simulink model "EVX_Lap_Simulation"  (R2018b)
settings: Solver=FixedStepAuto  StartTime=0  StopTime=100  FixedStep=0.01  MinStep=0.001  RelTol=1e-3
undefined symbols (not defined in the file): Car, dist, DOD, initial_velocity, motorefficiency, motormaxtorque, motorspeedradps, R0model, theta_d, Track_Dist, velocity_dnew, VoltageDOD, x, y
libraries: simulink x4
(part 1 of 3)
settings Model: Creator=Foster  LastModifiedBy=wjfos
settings SolverCC: AlgebraicLoopSolver=LineSearch
settings DebuggingCC: UnderspecifiedInitializationDetection=Classic  MergeDetectMultiDrivingBlocksExec=warning  MaxConsecutiveZCsMsg=warning  FcnCallInpInsideContextMsg=warning  UnconnectedInputMsg=none  UnconnectedOutputMsg=none  UnconnectedLineMsg=none  ModelReferenceExtraNoncontSigs=warning  UnderSpecifiedDimensionMsg=warning
settings HardwareCC: ProdBitPerLong=64  ProdHWDeviceType=Intel->x86-64 (Mac OS X)

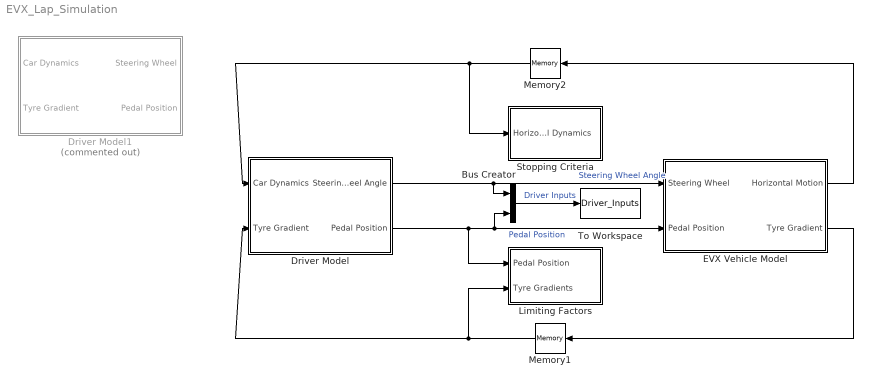
== system EVX_Lap_Simulation ==
  Bus Creator : BusCreator  Inputs=2
  Driver Model : Subsystem  Variant=on
  Driver Model1 : Subsystem  Commented=on
  EVX Vehicle Model : Subsystem
  Limiting Factors : Subsystem
  Memory1 : Memory  InheritSampleTime=on
  Memory2 : Memory  InheritSampleTime=on
  Stopping Criteria : Subsystem
  To Workspace : ToWorkspace  VariableName=Driver_Inputs  SaveFormat=Timeseries  SampleTime=-1
  wires:
  Driver Model/1(Steering Wheel Angle) -> Bus Creator/1, EVX Vehicle Model/1(Steering Wheel)  "Steering Wheel Angle"
  Driver Model/2(Pedal Position) -> Limiting Factors/1(Pedal Position), Bus Creator/2, EVX Vehicle Model/2(Pedal Position)  "Pedal Position"
  EVX Vehicle Model/1(Horizontal Motion) -> Memory2/1
  EVX Vehicle Model/2(Tyre Gradient) -> Memory1/1
  Memory1/1 -> Driver Model/2(Tyre Gradient), Limiting Factors/2(Tyre Gradients)
  Memory2/1 -> Driver Model/1(Car Dynamics), Stopping Criteria/1(Horizontal Dynamics)
  Bus Creator/1 -> To Workspace/1  "Driver Inputs"

== system EVX_Lap_Simulation/Driver Model ==
  Car Dynamics : Inport
  Tyre Gradient : Inport  Port=2
  Control System Driver Model : Subsystem  VariantControl=ControlSystemDriverModel
  Driver Input Model : Subsystem  VariantControl=InputDefinedDriverModel
  Steering Wheel Angle : Outport
  Pedal Position : Outport  Port=2

== system EVX_Lap_Simulation/Driver Model1 ==
  Car Dynamics : Inport
  Tyre Gradient : Inport  Port=2
  Control System Driver Model : Subsystem
  Driver Input Model : Subsystem
  Steering Wheel : Outport
  Pedal Position : Outport  Port=2

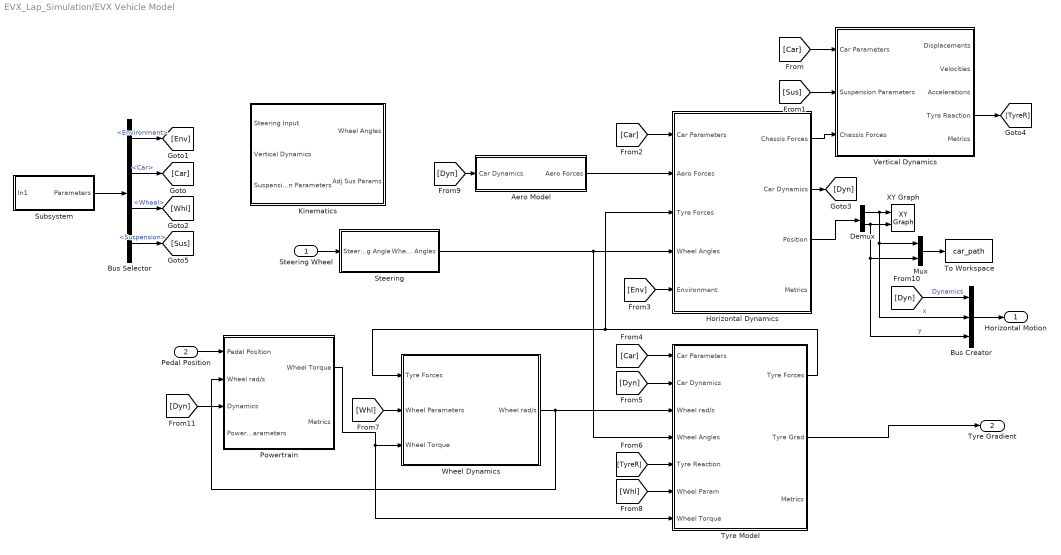
== system EVX_Lap_Simulation/EVX Vehicle Model ==
  Steering Wheel : Inport
  Pedal Position : Inport  Port=2
  Aero Model : Subsystem
  Bus Creator : BusCreator  Inputs=3
  Bus Selector : BusSelector  OutputSignals=Environment,Car,Wheel,Suspension
  Demux : Demux  Outputs=2
  Horizontal Dynamics : Subsystem
  Kinematics : Subsystem
  Mux : Mux  Inputs=2
  Powertrain : Subsystem
  Steering : Subsystem
  Subsystem : Subsystem
  To Workspace : ToWorkspace  VariableName=car_path  SaveFormat=Timeseries  SampleTime=-1
  Tyre Model : Subsystem
  Vertical Dynamics : Subsystem
  Wheel Dynamics : Subsystem
  XY Graph : simulink/Sinks/XY Graph  xmin=-400  xmax=100  ymin=-25  ymax=250  st=-1
  Horizontal Motion : Outport
  Tyre Gradient : Outport  Port=2
  wires:
  [Car] -> Vertical Dynamics/1(Car Parameters)
  [Sus] -> Vertical Dynamics/2(Suspension Parameters)
  [Car] -> Horizontal Dynamics/1(Car Parameters)
  Horizontal Dynamics/3(Position) -> Demux/1
  Demux/1 -> Mux/1, Bus Creator/2, XY Graph/1  "x"
  Demux/2 -> Mux/2, Bus Creator/3, XY Graph/2  "y"
  Steering/1(Wheel Angles) -> Horizontal Dynamics/4(Wheel Angles), Tyre Model/4(Wheel Angles)
  [Env] -> Horizontal Dynamics/5(Environment)
  [Car] -> Tyre Model/1(Car Parameters)
  Horizontal Dynamics/2(Car Dynamics) -> [Dyn]
  [Dyn] -> Tyre Model/2(Car Dynamics)
  [TyreR] -> Tyre Model/5(Tyre Reaction)
  [Whl] -> Wheel Dynamics/2(Wheel Parameters)
  Powertrain/1(Wheel Torque) -> Tyre Model/7(Wheel Torque), Wheel Dynamics/3(Wheel Torque)
  [Whl] -> Tyre Model/6(Wheel Param)
  Subsystem/1(Parameters) -> Bus Selector/1
  Bus Selector/1 -> [Env]  "<Environment>"
  Bus Selector/2 -> [Car]  "<Car>"
  Bus Selector/3 -> [Whl]  "<Wheel>"
  Bus Selector/4 -> [Sus]  "<Suspension>"
  [Dyn] -> Aero Model/1(Car Dynamics)
  Aero Model/1(Aero Forces) -> Horizontal Dynamics/2(Aero Forces)
  Horizontal Dynamics/1(Chassis Forces) -> Vertical Dynamics/3(Chassis Forces)
  Vertical Dynamics/4(Tyre Reaction) -> [TyreR]
  Wheel Dynamics/1(Wheel rad/s) -> Powertrain/2(Wheel rad/s), Tyre Model/3(Wheel rad/s)
  Tyre Model/1(Tyre Forces) -> Wheel Dynamics/1(Tyre Forces), Horizontal Dynamics/3(Tyre Forces)
  [Dyn] -> Bus Creator/1  "Dynamics"
  Mux/1 -> To Workspace/1
  Bus Creator/1 -> Horizontal Motion/1
  Pedal Position/1 -> Powertrain/1(Pedal Position)
  Steering Wheel/1 -> Steering/1(Steering Angle)
  Tyre Model/2(Tyre Grad) -> Tyre Gradient/1
  [Dyn] -> Powertrain/3(Dynamics)

== system EVX_Lap_Simulation/Limiting Factors ==
  Pedal Position : Inport
  Tyre Gradients : Inport  Port=2
  Braking Limit : MATLAB Function  TreatAsAtomicUnit=on
  Bus Creator : BusCreator  Inputs=4
  Cornering Limit : MATLAB Function  TreatAsAtomicUnit=on
  MATLAB Function : MATLAB Function  TreatAsAtomicUnit=on
  Power Limit : MATLAB Function  TreatAsAtomicUnit=on
  Scope : Scope  NumInputPorts=5
  To Workspace : ToWorkspace  VariableName=Limits  SaveFormat=Structure With Time  SampleTime=-1
  Traction Limit : MATLAB Function  TreatAsAtomicUnit=on
  wires:
  Pedal Position/1 -> Braking Limit/1(Pedal), Traction Limit/1(Pedal), Power Limit/1(Pedal)
  Tyre Gradients/1 -> Cornering Limit/1(Tyre_Grad), Traction Limit/2(Tyre_Grad), Braking Limit/2(Tyre_Grad)
  Power Limit/1(Limit) -> Bus Creator/1, MATLAB Function/1(Power_Lim), Scope/1
  Traction Limit/1(Limit) -> Bus Creator/2, Scope/2, MATLAB Function/2(Trac_Lim)
  Braking Limit/1(Limit) -> Bus Creator/3, Scope/3, MATLAB Function/3(Brake_Lim)
  Cornering Limit/1(Limit) -> Bus Creator/4, Scope/4, MATLAB Function/4(Corner_Lim)
  MATLAB Function/1(Limit) -> Scope/5
  Bus Creator/1 -> To Workspace/1

== system EVX_Lap_Simulation/Stopping Criteria ==
  Horizontal Dynamics : Inport
  Bus Selector8 : BusSelector  OutputSignals=x,y,Dynamics.Displacements.d_x
  Clock2 : Clock
  Constant2 : Constant  Value=Track_Dist
  MATLAB Function8 : MATLAB Function  TreatAsAtomicUnit=on
  Stop Simulation : Stop
  wires:
  Constant2/1 -> MATLAB Function8/4(dist_end)
  Bus Selector8/3 -> MATLAB Function8/3(dist_cur)  "<d_x>"
  Horizontal Dynamics/1 -> Bus Selector8/1
  Bus Selector8/2 -> MATLAB Function8/2(y)  "<y>"
  MATLAB Function8/1(Stop) -> Stop Simulation/1
  Bus Selector8/1 -> MATLAB Function8/1(x)  "<x>"
  Clock2/1 -> MATLAB Function8/5(t)

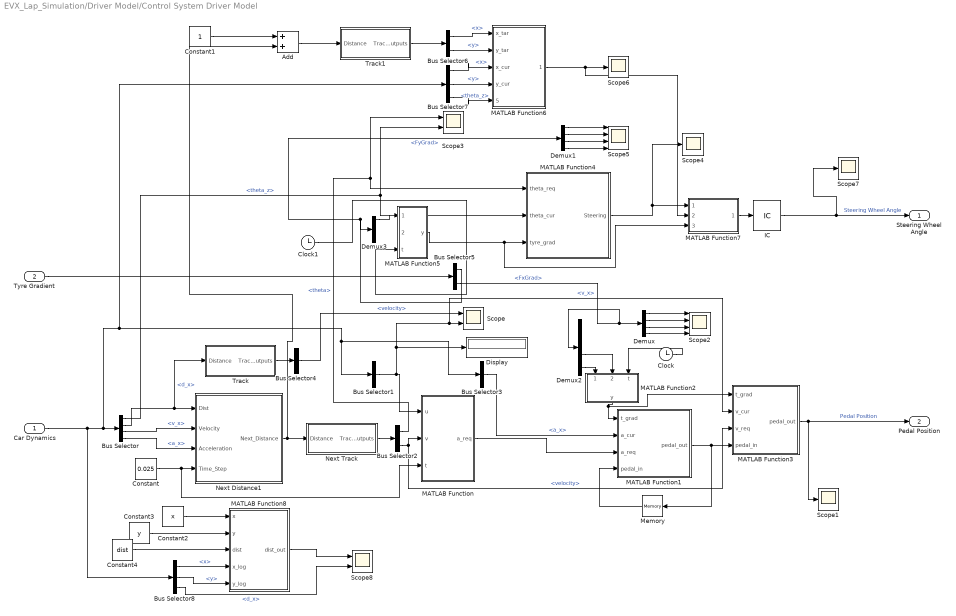
== system EVX_Lap_Simulation/Driver Model/Control System Driver Model ==
  Car Dynamics : Inport
  Tyre Gradient : Inport  Port=2
  Add : Sum
  Bus Selector : BusSelector  OutputSignals=Dynamics.Displacements.theta_z,Dynamics.Displacements.d_x,Dynamics.Velocities.v_x,Dynamics.Accelerations.a_x
  Bus Selector1 : BusSelector  OutputSignals=Dynamics.Velocities.v_x
  Bus Selector2 : BusSelector  OutputSignals=theta,velocity
  Bus Selector3 : BusSelector  OutputSignals=Dynamics.Accelerations.a_x
  Bus Selector4 : BusSelector  OutputSignals=velocity
  Bus Selector5 : BusSelector  OutputSignals=FyGrad,FxGrad
  Bus Selector6 : BusSelector  OutputSignals=x,y
  Bus Selector7 : BusSelector  OutputSignals=x,y,Dynamics.Displacements.theta_z
  Bus Selector8 : BusSelector  OutputSignals=x,y,Dynamics.Displacements.d_x
  Clock : Clock
  Clock1 : Clock
  Constant : Constant  Value=0.025
  Constant1 : Constant
  Constant2 : Constant  Value=x
  Constant3 : Constant  Value=y
  Constant4 : Constant  Value=dist
  Demux{,1..3} (4 alike) : Demux
  Display : Display
  IC : InitialCondition  Value=0
  MATLAB Function : MATLAB Function  TreatAsAtomicUnit=on
  MATLAB Function1 : MATLAB Function  TreatAsAtomicUnit=on
  MATLAB Function2 : MATLAB Function  TreatAsAtomicUnit=on
  MATLAB Function3 : MATLAB Function  TreatAsAtomicUnit=on
  MATLAB Function4 : MATLAB Function  TreatAsAtomicUnit=on
  MATLAB Function5 : MATLAB Function  TreatAsAtomicUnit=on
  MATLAB Function6 : MATLAB Function  TreatAsAtomicUnit=on
  MATLAB Function7 : MATLAB Function  TreatAsAtomicUnit=on
  MATLAB Function8 : MATLAB Function  TreatAsAtomicUnit=on
  Memory : Memory
  Next Distance1 : MATLAB Function  TreatAsAtomicUnit=on
  Next Track : Subsystem
  Scope : Scope  NumInputPorts=2
  Scope{1,4,6..7} (4 alike) : Scope
  Scope2 : Scope  NumInputPorts=4
  Scope3 : Scope  NumInputPorts=2
  Scope5 : Scope  NumInputPorts=4
  Scope8 : Scope  NumInputPorts=2
  Track : Subsystem
  Track1 : Subsystem
  Steering Wheel Angle : Outport
  Pedal Position : Outport  Port=2
  wires:
  MATLAB Function4/1(Steering) -> MATLAB Function7/1(steering_in), Scope4/1
  Bus Selector5/2 -> Demux2/1, Demux/1  "<FxGrad>"
  Next Track/1(Track Outputs) -> Bus Selector2/1
  Car Dynamics/1 -> Bus Selector8/1, Bus Selector7/1, Bus Selector3/1, Bus Selector1/1, Bus Selector/1
  Demux/2 -> Scope2/2
  MATLAB Function1/1(pedal_out) -> Memory/1, MATLAB Function3/4(pedal_in)
  Bus Selector4/1 -> Scope/1  "<velocity>"
  Demux2/3 -> MATLAB Function2/2(Fx_Grad_RR)
  Bus Selector1/1 -> Display/1, MATLAB Function3/2(v_cur), Scope/2, MATLAB Function/1(u)  "<v_x>"
  Next Distance1/1(Next_Distance) -> Next Track/1(Distance), Add/2
  Memory/1 -> MATLAB Function1/4(pedal_in)
  Constant1/1 -> Add/1
  MATLAB Function2/1(y) -> MATLAB Function1/1(t_grad), MATLAB Function3/1(t_grad)
  Bus Selector6/2 -> MATLAB Function6/2(y_tar)  "<y>"
  Bus Selector/1 -> Scope3/2, MATLAB Function4/2(theta_cur)  "<theta_z>"
  Constant/1 -> MATLAB Function/3(t), Next Distance1/4(Time_Step)
  IC/1 -> Steering Wheel Angle/1, Scope7/1  "Steering Wheel Angle"
  Bus Selector2/1 -> Scope3/1, MATLAB Function4/1(theta_req)  "<theta>"
  Bus Selector5/1 -> Demux3/1, Demux1/1  "<FyGrad>"
  Clock1/1 -> MATLAB Function5/3(t)
  Clock/1 -> MATLAB Function2/3(t)
  Track/1(Track Outputs) -> Bus Selector4/1
  Add/1 -> Track1/1(Distance)
  Demux/3 -> Scope2/3
  MATLAB Function3/1(pedal_out) -> Pedal Position/1, Scope1/1  "Pedal Position"
  Demux/1 -> Scope2/1
  Bus Selector/4 -> Next Distance1/3(Acceleration)  "<a_x>"
  Demux/4 -> Scope2/4
  MATLAB Function6/1(theta_error) -> MATLAB Function7/2(correction), Scope6/1
  Demux1/3 -> Scope5/3
  Bus Selector2/2 -> MATLAB Function/2(v), MATLAB Function3/3(v_req)  "<velocity>"
  Demux3/1 -> MATLAB Function5/1(Fy_Grad_FL)
  Bus Selector6/1 -> MATLAB Function6/1(x_tar)  "<x>"
  Demux1/2 -> Scope5/2
  MATLAB Function7/1(steering) -> IC/1
  Demux1/4 -> Scope5/4
  Demux2/4 -> MATLAB Function2/1(Fx_Grad_RL)
  Bus Selector7/2 -> MATLAB Function6/4(y_cur)  "<y>"
  Bus Selector7/1 -> MATLAB Function6/3(x_cur)  "<x>"
  MATLAB Function5/1(y) -> MATLAB Function7/3(Tyre_grad), MATLAB Function4/3(tyre_grad)
  MATLAB Function/1(a_req) -> MATLAB Function1/3(a_req)
  Bus Selector3/1 -> MATLAB Function1/2(a_cur)  "<a_x>"
  Track1/1(Track Outputs) -> Bus Selector6/1
  Bus Selector/3 -> Next Distance1/2(Velocity)  "<v_x>"
  Bus Selector7/3 -> MATLAB Function6/5(theta_cur)  "<theta_z>"
  Demux1/1 -> Scope5/1
  Tyre Gradient/1 -> Bus Selector5/1
  Constant2/1 -> MATLAB Function8/1(x)
  Constant3/1 -> MATLAB Function8/2(y)
  Constant4/1 -> MATLAB Function8/3(dist)
  Bus Selector8/1 -> MATLAB Function8/4(x_log)  "<x>"
  Bus Selector8/2 -> MATLAB Function8/5(y_log)  "<y>"
  Bus Selector8/3 -> Scope8/2  "<d_x>"
  MATLAB Function8/1(dist_out) -> Scope8/1
  Bus Selector/2 -> Track/1(Distance), Next Distance1/1(Dist)  "<d_x>"

== system EVX_Lap_Simulation/Driver Model/Driver Input Model ==
  From Workspace : FromWorkspace  VariableName=Steering_run  SampleTime=0
  From Workspace1 : FromWorkspace  VariableName=Pedal_run  SampleTime=0
  Steering Wheel Angle : Outport
  Pedal Position : Outport  Port=2
  wires:
  From Workspace1/1 -> Pedal Position/1
  From Workspace/1 -> Steering Wheel Angle/1

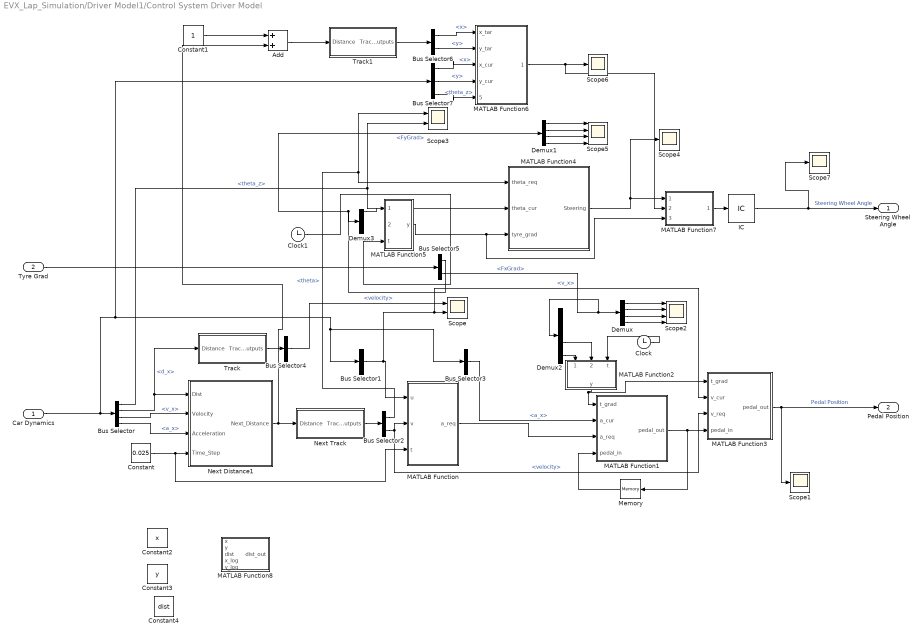
== system EVX_Lap_Simulation/Driver Model1/Control System Driver Model ==
  Car Dynamics : Inport
  Tyre Grad : Inport  Port=2
  Add : Sum
  Bus Selector : BusSelector  OutputSignals=Dynamics.Displacements.theta_z,Dynamics.Displacements.d_x,Dynamics.Velocities.v_x,Dynamics.Accelerations.a_x
  Bus Selector1 : BusSelector  OutputSignals=Dynamics.Velocities.v_x
  Bus Selector2 : BusSelector  OutputSignals=theta,velocity
  Bus Selector3 : BusSelector  OutputSignals=Dynamics.Accelerations.a_x
  Bus Selector4 : BusSelector  OutputSignals=velocity
  Bus Selector5 : BusSelector  OutputSignals=FyGrad,FxGrad
  Bus Selector6 : BusSelector  OutputSignals=x,y
  Bus Selector7 : BusSelector  OutputSignals=x,y,Dynamics.Displacements.theta_z
  Clock : Clock
  Clock1 : Clock
  Constant : Constant  Value=0.025
  Constant1 : Constant
  Constant2 : Constant  Value=x
  Constant3 : Constant  Value=y
  Constant4 : Constant  Value=dist
  Demux{,1..3} (4 alike) : Demux
  IC : InitialCondition  Value=0
  MATLAB Function : MATLAB Function  TreatAsAtomicUnit=on
  MATLAB Function1 : MATLAB Function  TreatAsAtomicUnit=on
  MATLAB Function2 : MATLAB Function  TreatAsAtomicUnit=on
  MATLAB Function3 : MATLAB Function  TreatAsAtomicUnit=on
  MATLAB Function4 : MATLAB Function  TreatAsAtomicUnit=on
  MATLAB Function5 : MATLAB Function  TreatAsAtomicUnit=on
  MATLAB Function6 : MATLAB Function  TreatAsAtomicUnit=on
  MATLAB Function7 : MATLAB Function  TreatAsAtomicUnit=on
  MATLAB Function8 : MATLAB Function  TreatAsAtomicUnit=on
  Memory : Memory
  Next Distance1 : MATLAB Function  TreatAsAtomicUnit=on
  Next Track : Subsystem
  Scope : Scope  NumInputPorts=2
  Scope{1,4,6..7} (4 alike) : Scope
  Scope2 : Scope  NumInputPorts=4
  Scope3 : Scope  NumInputPorts=2
  Scope5 : Scope  NumInputPorts=4
  Track : Subsystem
  Track1 : Subsystem
  Steering Wheel Angle : Outport
  Pedal Position : Outport  Port=2
  wires:
  MATLAB Function4/1(Steering) -> MATLAB Function7/1(steering_in), Scope4/1
  Bus Selector5/2 -> Demux2/1, Demux/1  "<FxGrad>"
  Next Track/1(Track Outputs) -> Bus Selector2/1
  Car Dynamics/1 -> Bus Selector7/1, Bus Selector3/1, Bus Selector1/1, Bus Selector/1
  Demux/2 -> Scope2/2
  MATLAB Function1/1(pedal_out) -> Memory/1, MATLAB Function3/4(pedal_in)
  Bus Selector4/1 -> Scope/1  "<velocity>"
  Demux2/3 -> MATLAB Function2/2(Fx_Grad_RR)
  Bus Selector1/1 -> MATLAB Function3/2(v_cur), Scope/2, MATLAB Function/1(u)  "<v_x>"
  Next Distance1/1(Next_Distance) -> Next Track/1(Distance), Add/2
  Memory/1 -> MATLAB Function1/4(pedal_in)
  Constant1/1 -> Add/1
  MATLAB Function2/1(y) -> MATLAB Function1/1(t_grad), MATLAB Function3/1(t_grad)
  Bus Selector/2 -> Next Distance1/1(Dist), Track/1(Distance)  "<d_x>"
  Bus Selector6/2 -> MATLAB Function6/2(y_tar)  "<y>"
  Bus Selector/1 -> Scope3/2, MATLAB Function4/2(theta_cur)  "<theta_z>"
  Constant/1 -> MATLAB Function/3(t), Next Distance1/4(Time_Step)
  IC/1 -> Steering Wheel Angle/1, Scope7/1  "Steering Wheel Angle"
  Bus Selector2/1 -> Scope3/1, MATLAB Function4/1(theta_req)  "<theta>"
  Bus Selector5/1 -> Demux3/1, Demux1/1  "<FyGrad>"
  Clock1/1 -> MATLAB Function5/3(t)
  Clock/1 -> MATLAB Function2/3(t)
  Track/1(Track Outputs) -> Bus Selector4/1
  Add/1 -> Track1/1(Distance)
  Demux/3 -> Scope2/3
  MATLAB Function3/1(pedal_out) -> Pedal Position/1, Scope1/1  "Pedal Position"
  Demux/1 -> Scope2/1
  Bus Selector/4 -> Next Distance1/3(Acceleration)  "<a_x>"
  Demux/4 -> Scope2/4
  MATLAB Function6/1(theta_error) -> MATLAB Function7/2(correction), Scope6/1
  Demux1/3 -> Scope5/3
  Bus Selector2/2 -> MATLAB Function/2(v), MATLAB Function3/3(v_req)  "<velocity>"
  Demux3/1 -> MATLAB Function5/1(Fy_Grad_FL)
  Bus Selector6/1 -> MATLAB Function6/1(x_tar)  "<x>"
  Demux1/2 -> Scope5/2
  MATLAB Function7/1(steering) -> IC/1
  Demux1/4 -> Scope5/4
  Demux2/4 -> MATLAB Function2/1(Fx_Grad_RL)
  Bus Selector7/2 -> MATLAB Function6/4(y_cur)  "<y>"
  Bus Selector7/1 -> MATLAB Function6/3(x_cur)  "<x>"
  MATLAB Function5/1(y) -> MATLAB Function7/3(Tyre_grad), MATLAB Function4/3(tyre_grad)
  MATLAB Function/1(a_req) -> MATLAB Function1/3(a_req)
  Bus Selector3/1 -> MATLAB Function1/2(a_cur)  "<a_x>"
  Track1/1(Track Outputs) -> Bus Selector6/1
  Bus Selector/3 -> Next Distance1/2(Velocity)  "<v_x>"
  Bus Selector7/3 -> MATLAB Function6/5(theta_cur)  "<theta_z>"
  Demux1/1 -> Scope5/1
  Tyre Grad/1 -> Bus Selector5/1

== system EVX_Lap_Simulation/Driver Model1/Driver Input Model ==
  In1 : Inport
  Out1 : Outport
  wires:
  In1/1 -> Out1/1

== system EVX_Lap_Simulation/EVX Vehicle Model/Aero Model ==
  Car Dynamics : Inport
  Bus Creator : BusCreator  Inputs=2
  Bus Creator1 : BusCreator  Inputs=2
  Bus Creator2 : BusCreator  Inputs=2
  Bus Selector : BusSelector  OutputSignals=Velocities.v_x
  Forces : MATLAB Function  TreatAsAtomicUnit=on
  Position : MATLAB Function  TreatAsAtomicUnit=on
  Aero Forces : Outport
  wires:
  Car Dynamics/1 -> Bus Selector/1
  Bus Selector/1 -> Forces/1(v_x), Position/1(v_x)  "<v_x>"
  Forces/1(F_L) -> Bus Creator/1
  Forces/2(F_D) -> Bus Creator/2
  Position/1(L) -> Bus Creator1/1
  Position/2(D) -> Bus Creator1/2
  Bus Creator/1 -> Bus Creator2/1  "Forces"
  Bus Creator1/1 -> Bus Creator2/2  "Position"
  Bus Creator2/1 -> Aero Forces/1

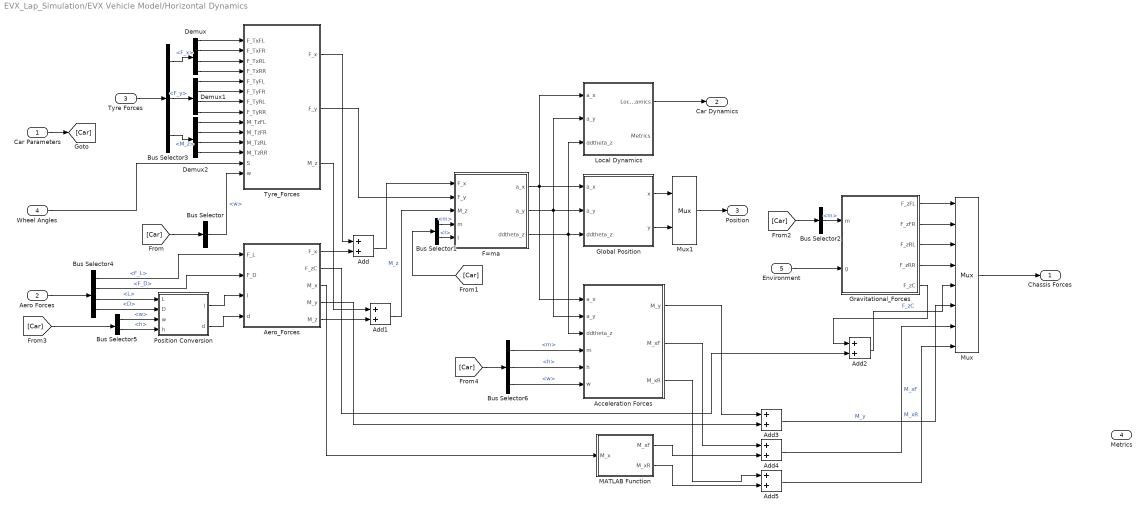
== system EVX_Lap_Simulation/EVX Vehicle Model/Horizontal Dynamics ==
  Car Parameters : Inport
  Aero Forces : Inport  Port=2
  Tyre Forces : Inport  Port=3
  Wheel Angles : Inport  Port=4
  Environment : Inport  Port=5
  Acceleration Forces : MATLAB Function  TreatAsAtomicUnit=on
  Add{,1..5} (6 alike) : Sum
  Aero_Forces : MATLAB Function  TreatAsAtomicUnit=on
  Bus Selector : BusSelector  OutputSignals=w
  Bus Selector1 : BusSelector  OutputSignals=m,I
  Bus Selector2 : BusSelector  OutputSignals=m
  Bus Selector3 : BusSelector  OutputSignals=F_x,F_y,M_z
  Bus Selector4 : BusSelector  OutputSignals=Forces.F_L,Forces.F_D,Position.L,Position.D
  Bus Selector5 : BusSelector  OutputSignals=w,h
  Bus Selector6 : BusSelector  OutputSignals=m,h,w
  Demux : Demux
  Demux1 : Demux
  Demux2 : Demux
  F=ma : MATLAB Function  TreatAsAtomicUnit=on
  Global Position : Subsystem
  Gravitational_Forces : MATLAB Function  TreatAsAtomicUnit=on
  Local Dynamics : Subsystem
  MATLAB Function : MATLAB Function  TreatAsAtomicUnit=on
  Mux : Mux  Inputs=8
      settings: DisplayOption=signals
  Mux1 : Mux  Inputs=2
      settings: DisplayOption=signals
  Position Conversion : MATLAB Function  TreatAsAtomicUnit=on
  Tyre_Forces : MATLAB Function  TreatAsAtomicUnit=on
  Chassis Forces : Outport
  Car Dynamics : Outport  Port=2
  Position : Outport  Port=3
  Metrics : Outport  Port=4
  wires:
  Car Parameters/1 -> [Car]
  [Car] -> Bus Selector/1
  Bus Selector/1 -> Tyre_Forces/14(w)  "<w>"
  Add2/1 -> Mux/5  "F_zC"
  Add1/1 -> F=ma/3(M_z)  "M_z"
  Add/1 -> F=ma/1(F_x)
  [Car] -> Bus Selector1/1
  Bus Selector1/1 -> F=ma/4(m)  "<m>"
  Bus Selector1/2 -> F=ma/5(I)  "<I>"
  F=ma/1(a_x) -> Local Dynamics/1(a_x), Global Position/1(a_x), Acceleration Forces/1(a_x)
  F=ma/2(a_y) -> Local Dynamics/2(a_y), Global Position/2(a_y), Acceleration Forces/2(a_y)
  F=ma/3(ddtheta_z) -> Local Dynamics/3(ddtheta_z), Global Position/3(ddtheta_z), Acceleration Forces/3(ddtheta_z)
  Bus Selector2/1 -> Gravitational_Forces/1(m)  "<m>"
  [Car] -> Bus Selector2/1
  Global Position/1(x) -> Mux1/1
  Global Position/2(y) -> Mux1/2
  Mux1/1 -> Position/1
  Environment/1 -> Gravitational_Forces/2(g)
  Local Dynamics/1(Local Dynamics) -> Car Dynamics/1
  Wheel Angles/1 -> Tyre_Forces/13(S)
  Aero Forces/1 -> Bus Selector4/1
  Bus Selector4/1 -> Aero_Forces/1(F_L)  "<F_L>"
  Bus Selector4/2 -> Aero_Forces/2(F_D)  "<F_D>"
  Bus Selector4/3 -> Position Conversion/1(L)  "<L>"
  Bus Selector4/4 -> Position Conversion/2(D)  "<D>"
  Position Conversion/1(l) -> Aero_Forces/3(l)
  Position Conversion/2(d) -> Aero_Forces/4(d)
  [Car] -> Bus Selector5/1
  Bus Selector5/1 -> Position Conversion/3(w)  "<w>"
  Bus Selector5/2 -> Position Conversion/4(h)  "<h>"
  Mux/1 -> Chassis Forces/1
  [Car] -> Bus Selector6/1
  Bus Selector6/1 -> Acceleration Forces/4(m)  "<m>"
  Bus Selector6/2 -> Acceleration Forces/5(h)  "<h>"
  Bus Selector6/3 -> Acceleration Forces/6(w)  "<w>"
  Gravitational_Forces/5(F_zC) -> Add2/1
  Gravitational_Forces/4(F_zRR) -> Mux/4
  Gravitational_Forces/3(F_zRL) -> Mux/3
  Gravitational_Forces/2(F_zFR) -> Mux/2
  Gravitational_Forces/1(F_zFL) -> Mux/1
  Aero_Forces/2(F_zC) -> Add2/2
  Aero_Forces/5(M_z) -> Add1/2
  Tyre_Forces/3(M_z) -> Add1/1
  Aero_Forces/1(F_x) -> Add/2
  Tyre_Forces/1(F_x) -> Add/1
  Tyre_Forces/2(F_y) -> F=ma/2(F_y)
  Aero_Forces/3(M_x) -> MATLAB Function/1(M_x)
  Aero_Forces/4(M_y) -> Add3/2
  Acceleration Forces/1(M_y) -> Add3/1
  Add3/1 -> Mux/6  "M_y"
  Acceleration Forces/2(M_xF) -> Add4/1
  MATLAB Function/1(M_xF) -> Add4/2
  Acceleration Forces/3(M_xR) -> Add5/1
  MATLAB Function/2(M_xR) -> Add5/2
  Add4/1 -> Mux/7  "M_xF"
  Add5/1 -> Mux/8  "M_xR"
  Tyre Forces/1 -> Bus Selector3/1
  Bus Selector3/1 -> Demux/1  "<F_x>"
  Bus Selector3/2 -> Demux1/1  "<F_y>"
  Bus Selector3/3 -> Demux2/1  "<M_z>"
  Demux/1 -> Tyre_Forces/1(F_TxFL)
  Demux/2 -> Tyre_Forces/2(F_TxFR)
  Demux/3 -> Tyre_Forces/3(F_TxRL)
  Demux/4 -> Tyre_Forces/4(F_TxRR)
  Demux1/1 -> Tyre_Forces/5(F_TyFL)
  Demux1/2 -> Tyre_Forces/6(F_TyFR)
  Demux1/3 -> Tyre_Forces/7(F_TyRL)
  Demux1/4 -> Tyre_Forces/8(F_TyRR)
  Demux2/1 -> Tyre_Forces/9(M_TzFL)
  Demux2/2 -> Tyre_Forces/10(M_TzFR)
  Demux2/3 -> Tyre_Forces/11(M_TzRL)
  Demux2/4 -> Tyre_Forces/12(M_TzRR)

== system EVX_Lap_Simulation/EVX Vehicle Model/Kinematics ==
  note: rear lookup table
  note: front lookup table
  Steering Input : Inport
  Vertical Dynamics : Inport  Port=2
  Suspension Parameters : Inport  Port=3
  Wheel Angles : Outport
  Adj Sus Params : Outport  Port=2

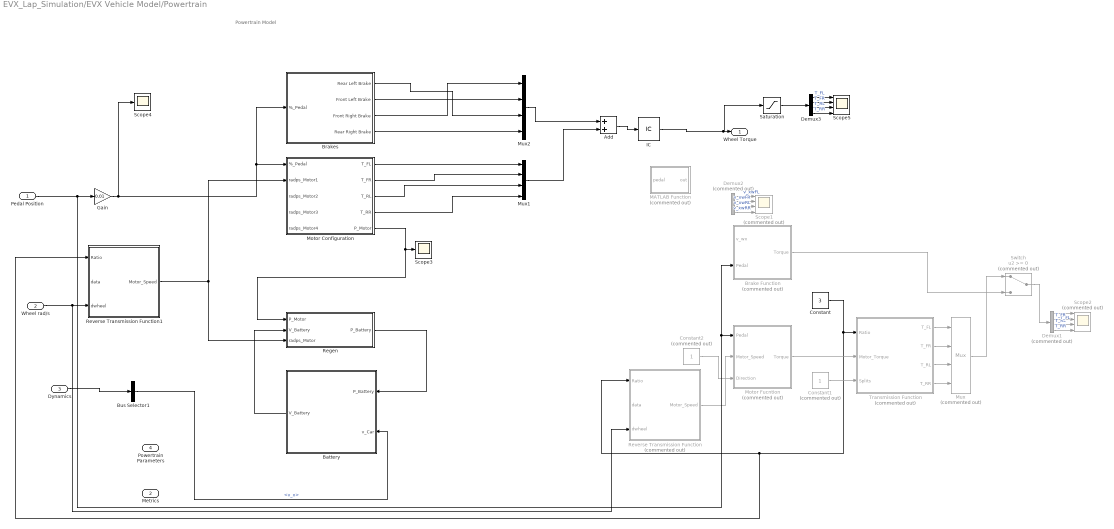
== system EVX_Lap_Simulation/EVX Vehicle Model/Powertrain ==
  note: Powertrain Model
  Pedal Position : Inport
  Wheel rad/s : Inport  Port=2
  Dynamics : Inport  Port=3
  Powertrain Parameters : Inport  Port=4
  Add : Sum
  Battery : Subsystem
      mask Display: image('C:\Users\v12st\OneDrive\Documents\ME4\FYP\Icons\Battery Icon.PNG');
  Brake Function : MATLAB Function  Commented=on  TreatAsAtomicUnit=on
  Brakes : Subsystem
      mask Display: image('C:\Users\v12st\OneDrive\Documents\ME4\FYP\Icons\BrakesIcon2.PNG');
  Bus Selector1 : BusSelector  OutputSignals=Velocities.v_x
  Constant : Constant  Value=3
  Constant1 : Constant  Commented=on
  Constant2 : Constant  Commented=on
  Demux1 : Demux  Commented=on
  Demux2 : Demux  Commented=on
  Demux3 : Demux
  Gain : Gain  Gain=0.01
  IC : InitialCondition  Value=0
  MATLAB Function : MATLAB Function  Commented=on  TreatAsAtomicUnit=on
  Motor Configuration : Subsystem  Variant=on
      mask Display: image('C:\Users\v12st\OneDrive\Documents\ME4\FYP\Icons\Motor Icon.PNG');
  Motor Fucntion : MATLAB Function  Commented=on  TreatAsAtomicUnit=on
  Mux : Mux  Commented=on
      settings: DisplayOption=signals
  Mux1 : Mux
  Mux2 : Mux
  Regen : Subsystem
  Reverse Transmission Function : MATLAB Function  Commented=on  TreatAsAtomicUnit=on
  Reverse Transmission Function1 : MATLAB Function  TreatAsAtomicUnit=on
  Saturation : Saturate  UpperLimit=Inf  LowerLimit=0
  Scope1 : Scope  Commented=on  NumInputPorts=4
  Scope2 : Scope  Commented=on  NumInputPorts=4
  Scope3 : Scope
  Scope4 : Scope
  Scope5 : Scope  NumInputPorts=4
  Switch : Switch  Commented=on
  Transmission Function : MATLAB Function  Commented=on  TreatAsAtomicUnit=on
  Wheel Torque : Outport
  Metrics : Outport  Port=2
  wires:
  Constant/1 -> Transmission Function/1(Ratio), Reverse Transmission Function1/1(Ratio), Reverse Transmission Function/1(Ratio)
  Constant1/1 -> Transmission Function/3(Splits)
  Reverse Transmission Function/1(Motor_Speed) -> Motor Fucntion/2(Motor_Speed)
  Mux/1 -> Switch/1
  Motor Fucntion/1(Torque) -> Transmission Function/2(Motor_Torque)
  Constant2/1 -> Motor Fucntion/3(Direction)
  Transmission Function/1(T_FL) -> Mux/1
  Transmission Function/2(T_FR) -> Mux/2
  Transmission Function/3(T_RL) -> Mux/3
  Transmission Function/4(T_RR) -> Mux/4
  Demux1/4 -> Scope2/4  "T_RR"
  Demux1/3 -> Scope2/3  "T_RL"
  Demux1/1 -> Scope2/1  "T_FL"
  Demux1/2 -> Scope2/2  "T_FR"
  Brake Function/1(Torque) -> Switch/3
  Demux2/2 -> Scope1/2  "v_xwFR"
  Demux2/1 -> Scope1/1  "v_xwFL"
  Demux2/4 -> Scope1/4  "v_xwRR"
  Demux2/3 -> Scope1/3  "v_xwRL"
  Switch/1 -> Demux1/1
  Motor Configuration/2(T_FR) -> Mux1/2
  Battery/1(V_Battery) -> Regen/2(V_Battery)
  Motor Configuration/3(T_RL) -> Mux1/3
  Motor Configuration/4(T_RR) -> Mux1/4
  Motor Configuration/1(T_FL) -> Mux1/1
  Regen/1(P_Battery) -> Battery/1(P_Battery)
  Pedal Position/1 -> Brake Function/2(Pedal), Motor Fucntion/1(Pedal), Gain/1
  Dynamics/1 -> Bus Selector1/1
  Wheel rad/s/1 -> Reverse Transmission Function/3(dwheel), Reverse Transmission Function1/3(dwheel)
  Reverse Transmission Function1/1(Motor_Speed) -> Regen/3(radps_Motor), Motor Configuration/2(radps_Motor1)
  Brakes/3(Front Right Brake) -> Mux2/1
  Brakes/2(Front Left Brake) -> Mux2/2
  Brakes/1(Rear Left Brake) -> Mux2/3
  Brakes/4(Rear Right Brake) -> Mux2/4
  Motor Configuration/5(P_Motor) -> Regen/1(P_Motor), Scope3/1
  Bus Selector1/1 -> Battery/2(v_Car)  "<v_x>"
  Mux1/1 -> Add/2
  Add/1 -> IC/1
  Gain/1 -> Scope4/1, Brakes/1(%_Pedal), Motor Configuration/1(%_Pedal)
  Mux2/1 -> Add/1
  IC/1 -> Saturation/1, Wheel Torque/1
  Demux3/2 -> Scope5/2  "T_FR"
  Demux3/1 -> Scope5/1  "T_FL"
  Demux3/4 -> Scope5/4  "T_RR"
  Demux3/3 -> Scope5/3  "T_RL"
  Saturation/1 -> Demux3/1

== system EVX_Lap_Simulation/EVX Vehicle Model/Steering ==
  Steering Angle : Inport
  Constant : Constant  Value=2
  Constant1 : Constant  Value=1.5
  Front/Rear Split : MATLAB Function  TreatAsAtomicUnit=on
  MATLAB Function : MATLAB Function  TreatAsAtomicUnit=on
  MATLAB Function1 : MATLAB Function  TreatAsAtomicUnit=on
  Mux : Mux
  Wheel Angles : Outport
  wires:
  Steering Angle/1 -> Front/Rear Split/1(Angle)
  Front/Rear Split/1(Steering_F) -> MATLAB Function/1(Steering_F)
  Front/Rear Split/2(Steering_R) -> MATLAB Function1/1(Steering_R)
  Constant/1 -> MATLAB Function/2(Ratio)
  Constant1/1 -> MATLAB Function1/2(Ratio)
  Mux/1 -> Wheel Angles/1
  MATLAB Function/1(S_FL) -> Mux/1
  MATLAB Function/2(S_FR) -> Mux/2
  MATLAB Function1/1(S_RL) -> Mux/3
  MATLAB Function1/2(S_RR) -> Mux/4

== system EVX_Lap_Simulation/EVX Vehicle Model/Subsystem ==
  In1 : Inport
  Bus Creator : BusCreator  Inputs=6
  Bus Creator1 : BusCreator  Inputs=6
  Bus Creator2 : BusCreator  Inputs=2
  Bus Creator3 : BusCreator  Inputs=1
  Bus Creator4 : BusCreator  Inputs=4
  Car Parameters : MATLAB Function  TreatAsAtomicUnit=on
  Environment Parameters : MATLAB Function  TreatAsAtomicUnit=on
  Suspension Parameters : MATLAB Function  TreatAsAtomicUnit=on
  Wheel Parameters : MATLAB Function  TreatAsAtomicUnit=on
  Parameters : Outport
  wires:
  Suspension Parameters/4(ct) -> Bus Creator/4
  Suspension Parameters/5(cs) -> Bus Creator/5
  Suspension Parameters/1(kt) -> Bus Creator/1
  Suspension Parameters/3(kr) -> Bus Creator/3
  Bus Creator/1 -> Bus Creator4/4  "Suspension"
  Car Parameters/1(w) -> Bus Creator1/1
  Bus Creator2/1 -> Bus Creator4/3  "Wheel"
  Bus Creator1/1 -> Bus Creator4/2  "Car"
  Suspension Parameters/2(ks) -> Bus Creator/2
  Car Parameters/5(cc) -> Bus Creator1/5
  Wheel Parameters/2(I) -> Bus Creator2/2
  Car Parameters/3(I) -> Bus Creator1/3
  Suspension Parameters/6(cr) -> Bus Creator/6
  Car Parameters/2(m) -> Bus Creator1/2
  Car Parameters/4(kc) -> Bus Creator1/4
  Wheel Parameters/1(r) -> Bus Creator2/1
  Environment Parameters/1(g) -> Bus Creator3/1
  Bus Creator3/1 -> Bus Creator4/1  "Environment"
  Bus Creator4/1 -> Parameters/1
  Car Parameters/6(h) -> Bus Creator1/6

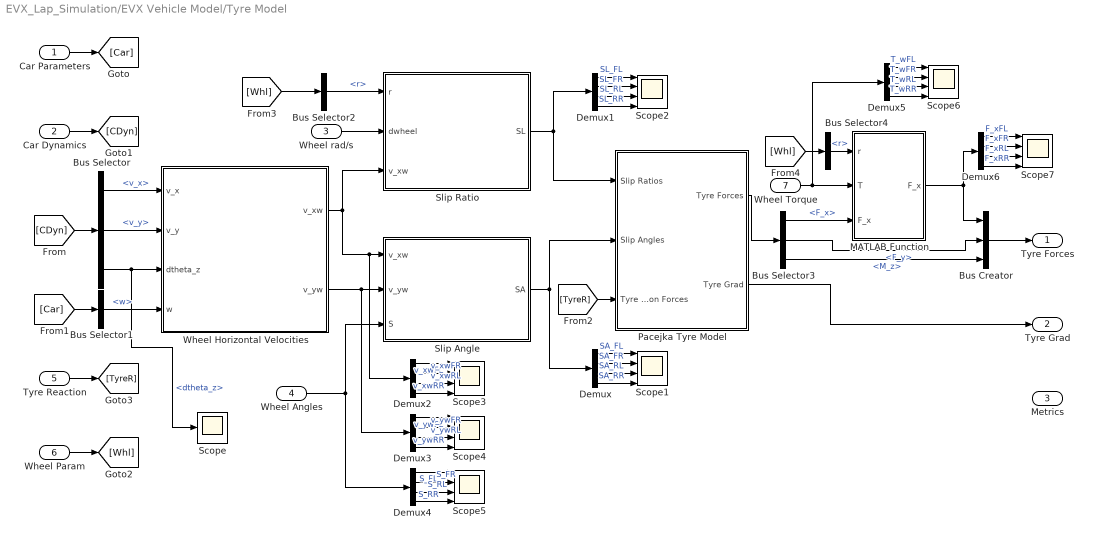
== system EVX_Lap_Simulation/EVX Vehicle Model/Tyre Model ==
  Car Parameters : Inport
  Car Dynamics : Inport  Port=2
  Wheel rad/s : Inport  Port=3
  Wheel Angles : Inport  Port=4
  Tyre Reaction : Inport  Port=5
  Wheel Param : Inport  Port=6
  Wheel Torque : Inport  Port=7
  Bus Creator : BusCreator  Inputs=3
  Bus Selector : BusSelector  OutputSignals=Velocities.v_x,Velocities.v_y,Velocities.dtheta_z
  Bus Selector1 : BusSelector  OutputSignals=w
  Bus Selector2 : BusSelector  OutputSignals=r
  Bus Selector3 : BusSelector  OutputSignals=F_x,F_y,M_z
  Bus Selector4 : BusSelector  OutputSignals=r
  Demux{,1..6} (7 alike) : Demux
  MATLAB Function : MATLAB Function  TreatAsAtomicUnit=on
  Pacejka Tyre Model : Subsystem
  Scope : Scope
  Scope{1..7} (7 alike) : Scope  NumInputPorts=4
  Slip Angle : MATLAB Function  TreatAsAtomicUnit=on
  Slip Ratio : MATLAB Function  TreatAsAtomicUnit=on
  Wheel Horizontal Velocities : MATLAB Function  TreatAsAtomicUnit=on
  Tyre Forces : Outport
  Tyre Grad : Outport  Port=2
  Metrics : Outport  Port=3
  wires:
  Car Parameters/1 -> [Car]
  Car Dynamics/1 -> [CDyn]
  Wheel rad/s/1 -> Slip Ratio/2(dwheel)
  [CDyn] -> Bus Selector/1
  Bus Selector/3 -> Scope/1, Wheel Horizontal Velocities/3(dtheta_z)  "<dtheta_z>"
  [Car] -> Bus Selector1/1
  Bus Selector1/1 -> Wheel Horizontal Velocities/4(w)  "<w>"
  Tyre Reaction/1 -> [TyreR]
  [TyreR] -> Pacejka Tyre Model/3(Tyre Reaction Forces)
  Slip Angle/1(SA) -> Demux/1, Pacejka Tyre Model/2(Slip Angles)
  Slip Ratio/1(SL) -> Demux1/1, Pacejka Tyre Model/1(Slip Ratios)
  Bus Selector/1 -> Wheel Horizontal Velocities/1(v_x)  "<v_x>"
  Bus Selector/2 -> Wheel Horizontal Velocities/2(v_y)  "<v_y>"
  Wheel Horizontal Velocities/1(v_xw) -> Slip Ratio/3(v_xw), Demux2/1, Slip Angle/1(v_xw)
  Wheel Horizontal Velocities/2(v_yw) -> Demux3/1, Slip Angle/2(v_yw)
  Wheel Angles/1 -> Slip Angle/3(S), Demux4/1
  Wheel Param/1 -> [Whl]
  [Whl] -> Bus Selector2/1
  Bus Selector2/1 -> Slip Ratio/1(r)  "<r>"
  Demux/1 -> Scope1/1  "SA_FL"
  Demux/2 -> Scope1/2  "SA_FR"
  Demux/3 -> Scope1/3  "SA_RL"
  Demux/4 -> Scope1/4  "SA_RR"
  Demux1/1 -> Scope2/1  "SL_FL"
  Demux1/2 -> Scope2/2  "SL_FR"
  Demux1/3 -> Scope2/3  "SL_RL"
  Demux1/4 -> Scope2/4  "SL_RR"
  Pacejka Tyre Model/1(Tyre Forces) -> Bus Selector3/1
  [Whl] -> Bus Selector4/1
  Bus Selector4/1 -> MATLAB Function/1(r)  "<r>"
  Wheel Torque/1 -> MATLAB Function/2(T), Demux5/1
  Bus Selector3/1 -> MATLAB Function/3("F_x ")  "<F_x>"
  MATLAB Function/1(F_x) -> Bus Creator/1, Demux6/1
  Bus Selector3/2 -> Bus Creator/2  "<F_y>"
  Bus Selector3/3 -> Bus Creator/3  "<M_z>"
  Bus Creator/1 -> Tyre Forces/1
  Demux2/4 -> Scope3/4  "v_xwRR"
  Demux2/1 -> Scope3/1  "v_xwFL"
  Demux2/3 -> Scope3/3  "v_xwRL"
  Demux2/2 -> Scope3/2  "v_xwFR"
  Demux3/4 -> Scope4/4  "v_ywRR"
  Demux3/1 -> Scope4/1  "v_ywFL"
  Demux3/3 -> Scope4/3  "v_ywRL"
  Demux3/2 -> Scope4/2  "v_ywFR"
  Demux4/4 -> Scope5/4  "S_RR"
  Demux4/1 -> Scope5/1  "S_FL"
  Demux4/3 -> Scope5/3  "S_RL"
  Demux4/2 -> Scope5/2  "S_FR"
  Demux5/3 -> Scope6/3  "T_wRL"
  Demux5/4 -> Scope6/4  "T_wRR"
  Demux5/1 -> Scope6/1  "T_wFL"
  Demux5/2 -> Scope6/2  "T_wFR"
  Demux6/3 -> Scope7/3  "F_xRL"
  Demux6/4 -> Scope7/4  "F_xRR"
  Demux6/1 -> Scope7/1  "F_xFL"
  Demux6/2 -> Scope7/2  "F_xFR"
  Pacejka Tyre Model/2(Tyre Grad) -> Tyre Grad/1

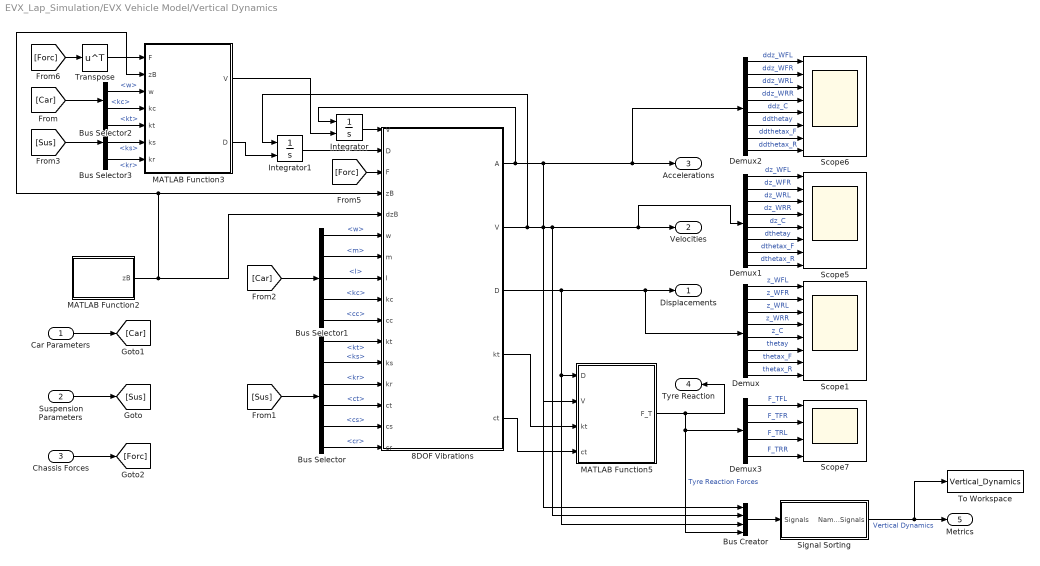
== system EVX_Lap_Simulation/EVX Vehicle Model/Vertical Dynamics ==
  Car Parameters : Inport
  Suspension Parameters : Inport  Port=2
  Chassis Forces : Inport  Port=3
  8DOF Vibrations : MATLAB Function  TreatAsAtomicUnit=on
  Bus Creator : BusCreator  Inputs=4
  Bus Selector : BusSelector  OutputSignals=kt,ks,kr,ct,cs,cr
  Bus Selector1 : BusSelector  OutputSignals=w,m,I,kc,cc
  Bus Selector2 : BusSelector  OutputSignals=w,kc
  Bus Selector3 : BusSelector  OutputSignals=kt,ks,kr
  Demux : Demux  Outputs=8
  Demux1 : Demux  Outputs=8
  Demux2 : Demux  Outputs=8
  Demux3 : Demux
  Integrator : Integrator  InitialConditionSource=external
  Integrator1 : Integrator  InitialConditionSource=external
  MATLAB Function2 : MATLAB Function  TreatAsAtomicUnit=on
  MATLAB Function3 : MATLAB Function  TreatAsAtomicUnit=on
  MATLAB Function5 : MATLAB Function  TreatAsAtomicUnit=on
  Scope1 : Scope  NumInputPorts=8
  Scope5 : Scope  NumInputPorts=8
  Scope6 : Scope  NumInputPorts=8
  Scope7 : Scope  NumInputPorts=4
  Signal Sorting : Subsystem
  To Workspace : ToWorkspace  VariableName=Vertical_Dynamics  SaveFormat=Timeseries  SampleTime=-1
  Transpose : Math  Operator=transpose  SaturateOnIntegerOverflow=on
  Displacements : Outport
  Velocities : Outport  Port=2
  Accelerations : Outport  Port=3
  Tyre Reaction : Outport  Port=4
  Metrics : Outport  Port=5
  wires:
  Demux/1 -> Scope1/1  "z_WFL"
  Demux/2 -> Scope1/2  "z_WFR"
  Demux/3 -> Scope1/3  "z_WRL"
  Demux/4 -> Scope1/4  "z_WRR"
  Demux/5 -> Scope1/5  "z_C"
  Demux/6 -> Scope1/6  "thetay"
  Demux/7 -> Scope1/7  "thetax_F"
  Demux/8 -> Scope1/8  "thetax_R"
  8DOF Vibrations/3(D) -> MATLAB Function5/1(D), Bus Creator/3, Demux/1, Displacements/1
  Demux1/1 -> Scope5/1  "dz_WFL"
  Demux1/3 -> Scope5/3  "dz_WRL"
  Demux1/2 -> Scope5/2  "dz_WFR"
  Demux1/4 -> Scope5/4  "dz_WRR"
  Demux1/8 -> Scope5/8  "dthetax_R"
  Demux1/6 -> Scope5/6  "dthetay"
  Demux1/5 -> Scope5/5  "dz_C"
  Demux1/7 -> Scope5/7  "dthetax_F"
  8DOF Vibrations/2(V) -> Velocities/1, Demux1/1, Bus Creator/2, MATLAB Function5/2(V), Integrator1/1
  Demux2/1 -> Scope6/1  "ddz_WFL"
  Demux2/3 -> Scope6/3  "ddz_WRL"
  Demux2/2 -> Scope6/2  "ddz_WFR"
  Demux2/4 -> Scope6/4  "ddz_WRR"
  Demux2/8 -> Scope6/8  "ddthetax_R"
  Demux2/6 -> Scope6/6  "ddthetay"
  Demux2/5 -> Scope6/5  "ddz_C"
  Demux2/7 -> Scope6/7  "ddthetax_F"
  8DOF Vibrations/1(A) -> Integrator/1, Accelerations/1, Demux2/1, Bus Creator/1
  Demux3/1 -> Scope7/1  "F_TFL"
  Demux3/3 -> Scope7/3  "F_TRL"
  Demux3/2 -> Scope7/2  "F_TFR"
  Demux3/4 -> Scope7/4  "F_TRR"
  8DOF Vibrations/4(kt) -> MATLAB Function5/3(kt)
  8DOF Vibrations/5(ct) -> MATLAB Function5/4(ct)
  MATLAB Function2/1(zB) -> 8DOF Vibrations/5(dzB), 8DOF Vibrations/4(zB), MATLAB Function3/2(zB)
  Integrator1/1 -> 8DOF Vibrations/2("D ")
  Integrator/1 -> 8DOF Vibrations/1("V ")
  Suspension Parameters/1 -> [Sus]
  Car Parameters/1 -> [Car]
  [Sus] -> Bus Selector/1
  Bus Selector/1 -> 8DOF Vibrations/11("kt ")  "<kt>"
  Bus Selector/2 -> 8DOF Vibrations/12(ks)  "<ks>"
  Bus Selector/3 -> 8DOF Vibrations/13(kr)  "<kr>"
  Bus Selector/4 -> 8DOF Vibrations/14("ct ")  "<ct>"
  Bus Selector/5 -> 8DOF Vibrations/15(cs)  "<cs>"
  Bus Selector/6 -> 8DOF Vibrations/16(cr)  "<cr>"
  [Car] -> Bus Selector1/1
  Bus Selector1/1 -> 8DOF Vibrations/6(w)  "<w>"
  Bus Selector1/2 -> 8DOF Vibrations/7(m)  "<m>"
  Bus Selector1/4 -> 8DOF Vibrations/9(kc)  "<kc>"
  Bus Selector1/5 -> 8DOF Vibrations/10(cc)  "<cc>"
  [Car] -> Bus Selector2/1
  Bus Selector2/1 -> MATLAB Function3/3(w)  "<w>"
  Bus Selector2/2 -> MATLAB Function3/4(kc)  "<kc>"
  [Sus] -> Bus Selector3/1
  Bus Selector3/1 -> MATLAB Function3/5(kt)  "<kt>"
  Bus Selector3/2 -> MATLAB Function3/6(ks)  "<ks>"
  Bus Selector3/3 -> MATLAB Function3/7(kr)  "<kr>"
  MATLAB Function5/1(F_T) -> Demux3/1, Bus Creator/4, Tyre Reaction/1  "Tyre Reaction Forces"
  MATLAB Function3/1(V) -> Integrator/2
  MATLAB Function3/2(D) -> Integrator1/2
  Bus Selector1/3 -> 8DOF Vibrations/8(I)  "<I>"
  Chassis Forces/1 -> [Forc]
  [Forc] -> 8DOF Vibrations/3(F)
  [Forc] -> Transpose/1
  Transpose/1 -> MATLAB Function3/1(F)
  Bus Creator/1 -> Signal Sorting/1(Signals)
  Signal Sorting/1(Named Signals) -> To Workspace/1, Metrics/1  "Vertical Dynamics"

== system EVX_Lap_Simulation/EVX Vehicle Model/Wheel Dynamics ==
  Tyre Forces : Inport
  Wheel Parameters : Inport  Port=2
  Wheel Torque : Inport  Port=3
  Bus Selector : BusSelector  OutputSignals=F_x
  Bus Selector1 : BusSelector  OutputSignals=I,r
  Integrator : Integrator  InitialConditionSource=external
  Mux : Mux
  Scope{,1..3} (4 alike) : Scope
  Scope4 : Scope  NumInputPorts=2
  Wheel Acceleration : MATLAB Function  TreatAsAtomicUnit=on
  WheelFL Initial : Constant  Value=initial_velocity/Car.Dimension.WheelFL.Radius
  WheelFR Initial : Constant  Value=initial_velocity/Car.Dimension.WheelFR.Radius
  WheelRL Initial : Constant  Value=initial_velocity/Car.Dimension.WheelRL.Radius
  WheelRR Initial : Constant  Value=initial_velocity/Car.Dimension.WheelRR.Radius
  Wheel rad/s : Outport
  wires:
  Wheel Acceleration/1(ddwheel) -> Scope4/1, Integrator/1
  Wheel Parameters/1 -> Bus Selector1/1
  Bus Selector1/1 -> Scope/1, Wheel Acceleration/3(I)  "<I>"
  Bus Selector1/2 -> Scope3/1, Wheel Acceleration/4(r)  "<r>"
  Tyre Forces/1 -> Bus Selector/1
  Bus Selector/1 -> Scope2/1, Wheel Acceleration/1(F_x)  "<F_x>"
  Wheel Torque/1 -> Scope1/1, Wheel Acceleration/2(T)
  Integrator/1 -> Scope4/2, Wheel rad/s/1
  Mux/1 -> Integrator/2
  WheelFL Initial/1 -> Mux/1
  WheelFR Initial/1 -> Mux/2
  WheelRL Initial/1 -> Mux/3
  WheelRR Initial/1 -> Mux/4

== system EVX_Lap_Simulation/Driver Model/Control System Driver Model/Next Track ==
  Distance : Inport
  Bus Creator : BusCreator  Inputs=4
  Theta : Lookup_n-D  NumberOfTableDimensions=1  BreakpointsForDimension1=dist  BreakpointsForDimension2=dist  BreakpointsForDimension3=dist  BreakpointsForDimension4=dist  Table=theta_d  ExtrapMethod=Clip  UseLastTableValue=on  InternalRulePriority=Speed  RndMeth=Simplest  InputSameDT=on
  Velocity : Lookup_n-D  NumberOfTableDimensions=1  BreakpointsForDimension1=dist  BreakpointsForDimension2=dist  BreakpointsForDimension3=dist  BreakpointsForDimension4=dist  Table=velocity_dnew  ExtrapMethod=Clip  UseLastTableValue=on  InternalRulePriority=Speed  RndMeth=Simplest  InputSameDT=on
  X : Lookup_n-D  NumberOfTableDimensions=1  BreakpointsForDimension1=dist  BreakpointsForDimension2=dist  BreakpointsForDimension3=dist  BreakpointsForDimension4=dist  Table=x  InternalRulePriority=Speed  RndMeth=Simplest  InputSameDT=on
  Y : Lookup_n-D  NumberOfTableDimensions=1  BreakpointsForDimension1=dist  BreakpointsForDimension2=dist  BreakpointsForDimension3=dist  BreakpointsForDimension4=dist  Table=y  InternalRulePriority=Speed  RndMeth=Simplest  InputSameDT=on
  Track Outputs : Outport
  wires:
  Distance/1 -> Velocity/1, Theta/1, Y/1, X/1
  X/1 -> Bus Creator/1  "x"
  Y/1 -> Bus Creator/2  "y"
  Theta/1 -> Bus Creator/3  "theta"
  Velocity/1 -> Bus Creator/4  "velocity"
  Bus Creator/1 -> Track Outputs/1

== system EVX_Lap_Simulation/Driver Model/Control System Driver Model/Track ==
  Distance : Inport
  Bus Creator : BusCreator  Inputs=4
  Theta : Lookup_n-D  NumberOfTableDimensions=1  BreakpointsForDimension1=dist  BreakpointsForDimension2=dist  BreakpointsForDimension3=dist  BreakpointsForDimension4=dist  Table=theta_d  ExtrapMethod=Clip  UseLastTableValue=on  InternalRulePriority=Speed  RndMeth=Simplest  InputSameDT=on
  Velocity : Lookup_n-D  NumberOfTableDimensions=1  BreakpointsForDimension1=dist  BreakpointsForDimension2=dist  BreakpointsForDimension3=dist  BreakpointsForDimension4=dist  Table=velocity_dnew  ExtrapMethod=Clip  UseLastTableValue=on  InternalRulePriority=Speed  RndMeth=Simplest  InputSameDT=on
  X : Lookup_n-D  NumberOfTableDimensions=1  BreakpointsForDimension1=dist  BreakpointsForDimension2=dist  BreakpointsForDimension3=dist  BreakpointsForDimension4=dist  Table=x  InternalRulePriority=Speed  RndMeth=Simplest  InputSameDT=on
  Y : Lookup_n-D  NumberOfTableDimensions=1  BreakpointsForDimension1=dist  BreakpointsForDimension2=dist  BreakpointsForDimension3=dist  BreakpointsForDimension4=dist  Table=y  InternalRulePriority=Speed  RndMeth=Simplest  InputSameDT=on
  Track Outputs : Outport
  wires:
  Distance/1 -> Velocity/1, Theta/1, Y/1, X/1
  X/1 -> Bus Creator/1  "x"
  Y/1 -> Bus Creator/2  "y"
  Theta/1 -> Bus Creator/3  "theta"
  Velocity/1 -> Bus Creator/4  "velocity"
  Bus Creator/1 -> Track Outputs/1

== system EVX_Lap_Simulation/Driver Model/Control System Driver Model/Track1 ==
  Distance : Inport
  Bus Creator : BusCreator  Inputs=4
  Theta : Lookup_n-D  NumberOfTableDimensions=1  BreakpointsForDimension1=dist  BreakpointsForDimension2=dist  BreakpointsForDimension3=dist  BreakpointsForDimension4=dist  Table=theta_d  InternalRulePriority=Speed  RndMeth=Simplest  InputSameDT=on
  Velocity : Lookup_n-D  NumberOfTableDimensions=1  BreakpointsForDimension1=dist  BreakpointsForDimension2=dist  BreakpointsForDimension3=dist  BreakpointsForDimension4=dist  Table=velocity_dnew  InternalRulePriority=Speed  RndMeth=Simplest  InputSameDT=on
  X : Lookup_n-D  NumberOfTableDimensions=1  BreakpointsForDimension1=dist  BreakpointsForDimension2=dist  BreakpointsForDimension3=dist  BreakpointsForDimension4=dist  Table=x  InternalRulePriority=Speed  RndMeth=Simplest  InputSameDT=on
  Y : Lookup_n-D  NumberOfTableDimensions=1  BreakpointsForDimension1=dist  BreakpointsForDimension2=dist  BreakpointsForDimension3=dist  BreakpointsForDimension4=dist  Table=y  InternalRulePriority=Speed  RndMeth=Simplest  InputSameDT=on
  Track Outputs : Outport
  wires:
  Distance/1 -> Velocity/1, Theta/1, Y/1, X/1
  X/1 -> Bus Creator/1  "x"
  Y/1 -> Bus Creator/2  "y"
  Theta/1 -> Bus Creator/3  "theta"
  Velocity/1 -> Bus Creator/4  "velocity"
  Bus Creator/1 -> Track Outputs/1

== system EVX_Lap_Simulation/Driver Model1/Control System Driver Model/Next Track ==
  Distance : Inport
  Bus Creator : BusCreator  Inputs=4
  Theta : Lookup_n-D  NumberOfTableDimensions=1  BreakpointsForDimension1=dist  BreakpointsForDimension2=dist  BreakpointsForDimension3=dist  BreakpointsForDimension4=dist  Table=theta_d  InternalRulePriority=Speed  RndMeth=Simplest  InputSameDT=on
  Velocity : Lookup_n-D  NumberOfTableDimensions=1  BreakpointsForDimension1=dist  BreakpointsForDimension2=dist  BreakpointsForDimension3=dist  BreakpointsForDimension4=dist  Table=velocity_dnew  InternalRulePriority=Speed  RndMeth=Simplest  InputSameDT=on
  X : Lookup_n-D  NumberOfTableDimensions=1  BreakpointsForDimension1=dist  BreakpointsForDimension2=dist  BreakpointsForDimension3=dist  BreakpointsForDimension4=dist  Table=x(1:end-1)  InternalRulePriority=Speed  RndMeth=Simplest  InputSameDT=on
  Y : Lookup_n-D  NumberOfTableDimensions=1  BreakpointsForDimension1=dist  BreakpointsForDimension2=dist  BreakpointsForDimension3=dist  BreakpointsForDimension4=dist  Table=y(1:end-1)  InternalRulePriority=Speed  RndMeth=Simplest  InputSameDT=on
  Track Outputs : Outport
  wires:
  Distance/1 -> Velocity/1, Theta/1, Y/1, X/1
  X/1 -> Bus Creator/1  "x"
  Y/1 -> Bus Creator/2  "y"
  Theta/1 -> Bus Creator/3  "theta"
  Velocity/1 -> Bus Creator/4  "velocity"
  Bus Creator/1 -> Track Outputs/1

== system EVX_Lap_Simulation/Driver Model1/Control System Driver Model/Track ==
  Distance : Inport
  Bus Creator : BusCreator  Inputs=4
  Theta : Lookup_n-D  NumberOfTableDimensions=1  BreakpointsForDimension1=dist  BreakpointsForDimension2=dist  BreakpointsForDimension3=dist  BreakpointsForDimension4=dist  Table=theta_d  InternalRulePriority=Speed  RndMeth=Simplest  InputSameDT=on
  Velocity : Lookup_n-D  NumberOfTableDimensions=1  BreakpointsForDimension1=dist  BreakpointsForDimension2=dist  BreakpointsForDimension3=dist  BreakpointsForDimension4=dist  Table=velocity_dnew  InternalRulePriority=Speed  RndMeth=Simplest  InputSameDT=on
  X : Lookup_n-D  NumberOfTableDimensions=1  BreakpointsForDimension1=dist  BreakpointsForDimension2=dist  BreakpointsForDimension3=dist  BreakpointsForDimension4=dist  Table=x(1:end-1)  InternalRulePriority=Speed  RndMeth=Simplest  InputSameDT=on
  Y : Lookup_n-D  NumberOfTableDimensions=1  BreakpointsForDimension1=dist  BreakpointsForDimension2=dist  BreakpointsForDimension3=dist  BreakpointsForDimension4=dist  Table=y(1:end-1)  InternalRulePriority=Speed  RndMeth=Simplest  InputSameDT=on
  Track Outputs : Outport
  wires:
  Distance/1 -> Velocity/1, Theta/1, Y/1, X/1
  X/1 -> Bus Creator/1  "x"
  Y/1 -> Bus Creator/2  "y"
  Theta/1 -> Bus Creator/3  "theta"
  Velocity/1 -> Bus Creator/4  "velocity"
  Bus Creator/1 -> Track Outputs/1

== system EVX_Lap_Simulation/Driver Model1/Control System Driver Model/Track1 ==
  Distance : Inport
  Bus Creator : BusCreator  Inputs=4
  Theta : Lookup_n-D  NumberOfTableDimensions=1  BreakpointsForDimension1=dist  BreakpointsForDimension2=dist  BreakpointsForDimension3=dist  BreakpointsForDimension4=dist  Table=theta_d  InternalRulePriority=Speed  RndMeth=Simplest  InputSameDT=on
  Velocity : Lookup_n-D  NumberOfTableDimensions=1  BreakpointsForDimension1=dist  BreakpointsForDimension2=dist  BreakpointsForDimension3=dist  BreakpointsForDimension4=dist  Table=velocity_dnew  InternalRulePriority=Speed  RndMeth=Simplest  InputSameDT=on
  X : Lookup_n-D  NumberOfTableDimensions=1  BreakpointsForDimension1=dist  BreakpointsForDimension2=dist  BreakpointsForDimension3=dist  BreakpointsForDimension4=dist  Table=x(1:end-1)  InternalRulePriority=Speed  RndMeth=Simplest  InputSameDT=on
  Y : Lookup_n-D  NumberOfTableDimensions=1  BreakpointsForDimension1=dist  BreakpointsForDimension2=dist  BreakpointsForDimension3=dist  BreakpointsForDimension4=dist  Table=y(1:end-1)  InternalRulePriority=Speed  RndMeth=Simplest  InputSameDT=on
  Track Outputs : Outport
  wires:
  Distance/1 -> Velocity/1, Theta/1, Y/1, X/1
  X/1 -> Bus Creator/1  "x"
  Y/1 -> Bus Creator/2  "y"
  Theta/1 -> Bus Creator/3  "theta"
  Velocity/1 -> Bus Creator/4  "velocity"
  Bus Creator/1 -> Track Outputs/1

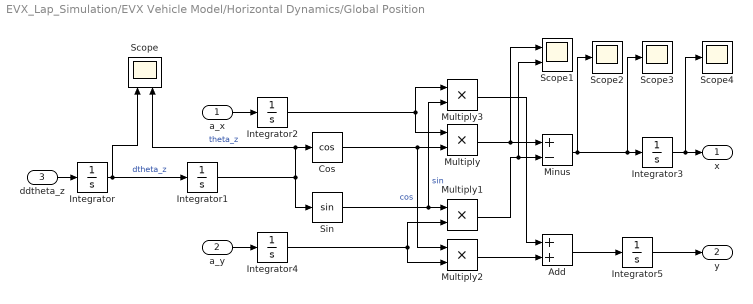
== system EVX_Lap_Simulation/EVX Vehicle Model/Horizontal Dynamics/Global Position ==
  a_x : Inport
  a_y : Inport  Port=2
  ddtheta_z : Inport  Port=3
  Add : Sum
  Cos : Trigonometry  Operator=cos
  Integrator : Integrator
  Integrator1 : Integrator  InitialCondition=theta_d(1)
  Integrator2 : Integrator  InitialCondition=initial_velocity
  Integrator3 : Integrator  InitialCondition=x(1)
  Integrator4 : Integrator
  Integrator5 : Integrator  InitialCondition=y(1)
  Minus : Sum  Inputs=+-
  Multiply{,1..3} (4 alike) : Product
  Scope : Scope  NumInputPorts=2
  Scope1 : Scope  NumInputPorts=2
  Scope2 : Scope
  Scope3 : Scope
  Scope4 : Scope
  Sin : Trigonometry
  x : Outport
  y : Outport  Port=2
  wires:
  ddtheta_z/1 -> Integrator/1
  Integrator/1 -> Scope/1, Integrator1/1  "dtheta_z"
  Integrator1/1 -> Scope/2, Cos/1, Sin/1  "theta_z"
  a_x/1 -> Integrator2/1
  Cos/1 -> Multiply2/1, Multiply/2  "cos"
  Sin/1 -> Multiply3/2, Multiply1/1  "sin"
  a_y/1 -> Integrator4/1
  Multiply/1 -> Scope1/1, Minus/1
  Multiply1/1 -> Scope1/2, Minus/2
  Multiply2/1 -> Add/2
  Multiply3/1 -> Add/1
  Minus/1 -> Scope3/1, Integrator3/1, Scope2/1
  Integrator3/1 -> Scope4/1, x/1
  Add/1 -> Integrator5/1
  Integrator4/1 -> Multiply2/2, Multiply1/2
  Integrator5/1 -> y/1
  Integrator2/1 -> Multiply/1, Multiply3/1

== system EVX_Lap_Simulation/EVX Vehicle Model/Horizontal Dynamics/Local Dynamics ==
  a_x : Inport
  a_y : Inport  Port=2
  ddtheta_z : Inport  Port=3
  Bus Creator{,1..3} (4 alike) : BusCreator  Inputs=3
  Integrator : Integrator  InitialCondition=initial_velocity
  Integrator{1..4} (4 alike) : Integrator
  Integrator5 : Integrator  InitialCondition=theta_d(1)
  Scope : Scope
  Subsystem : Subsystem
  To Workspace : ToWorkspace  VariableName=dist_log  SaveFormat=Timeseries  SampleTime=-1
  To Workspace1 : ToWorkspace  VariableName=Horizontal_Dynamics  SaveFormat=Timeseries  SampleTime=-1
  Local Dynamics : Outport
  Metrics : Outport  Port=2
  wires:
  Integrator/1 -> Bus Creator1/1, Integrator3/1  "v_x"
  Integrator2/1 -> Bus Creator1/3, Integrator5/1  "dtheta_z"
  Integrator1/1 -> Bus Creator1/2, Integrator4/1  "v_y"
  a_x/1 -> Bus Creator/1, Integrator/1  "a_x"
  a_y/1 -> Bus Creator/2, Integrator1/1  "a_y"
  ddtheta_z/1 -> Bus Creator/3, Integrator2/1  "ddtheta_z"
  Integrator4/1 -> Bus Creator2/2  "d_y"
  Integrator3/1 -> To Workspace/1, Bus Creator2/1  "d_x"
  Integrator5/1 -> Scope/1, Bus Creator2/3  "theta_z"
  Bus Creator1/1 -> Bus Creator3/2  "Velocities"
  Bus Creator/1 -> Bus Creator3/1  "Accelerations"
  Bus Creator2/1 -> Bus Creator3/3  "Displacements"
  Bus Creator3/1 -> Subsystem/1(Signals), Local Dynamics/1  "Horizontal Dynamics"
  Subsystem/1(Named Signals) -> To Workspace1/1, Metrics/1  "Horizontal Dynamics"

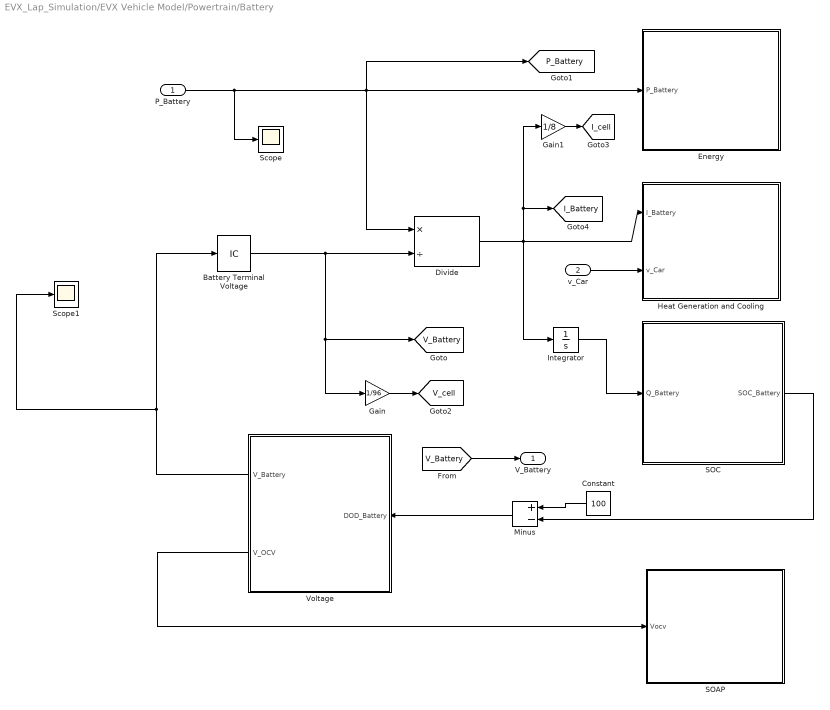
== system EVX_Lap_Simulation/EVX Vehicle Model/Powertrain/Battery ==
  P_Battery : Inport
  v_Car : Inport  Port=2
  Battery Terminal Voltage : InitialCondition  Value=405
  Constant : Constant  Value=100
  Divide : Product  Inputs=*/
  Energy : Subsystem
  Gain : Gain  Gain=1/96
  Gain1 : Gain  Gain=1/8
  Heat Generation and Cooling : Subsystem
  Integrator : Integrator
  Minus : Sum  Inputs=+-
  SOAP : Subsystem
  SOC : Subsystem
  Scope : Scope
  Scope1 : Scope
  Voltage : Subsystem
  V_Battery : Outport
  tag scope: I_Battery=global, I_cell=global, P_Battery=global, V_Battery=global, V_cell=global
  wires:
  P_Battery/1 -> Scope/1, [P_Battery], Divide/1, Energy/1(P_Battery)
  Integrator/1 -> SOC/1(Q_Battery)
  Battery Terminal Voltage/1 -> Divide/2, Gain/1, [V_Battery]
  [V_Battery] -> V_Battery/1
  Divide/1 -> Integrator/1, Gain1/1, [I_Battery], Heat Generation and Cooling/1(I_Battery)
  Voltage/2(V_OCV) -> SOAP/1(Vocv)
  Voltage/1(V_Battery) -> Scope1/1, Battery Terminal Voltage/1
  Gain/1 -> [V_cell]
  Gain1/1 -> [I_cell]
  v_Car/1 -> Heat Generation and Cooling/2(v_Car)
  Constant/1 -> Minus/1
  SOC/1(SOC_Battery) -> Minus/2
  Minus/1 -> Voltage/1(DOD_Battery)
